simulink model "lazo_abierto"  (R2021b)
settings: Solver=VariableStepAuto  StartTime=0.0  StopTime=500  RelTol=1e-3
settings Model: Creator=sebas  LastModifiedBy=sebas

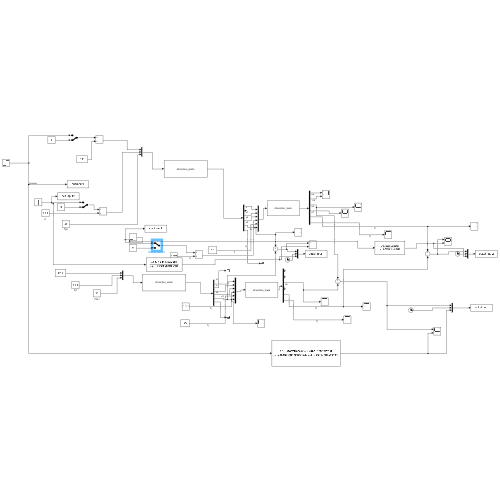
[thumbnail: Simulink's stored preview of the top-level diagram]
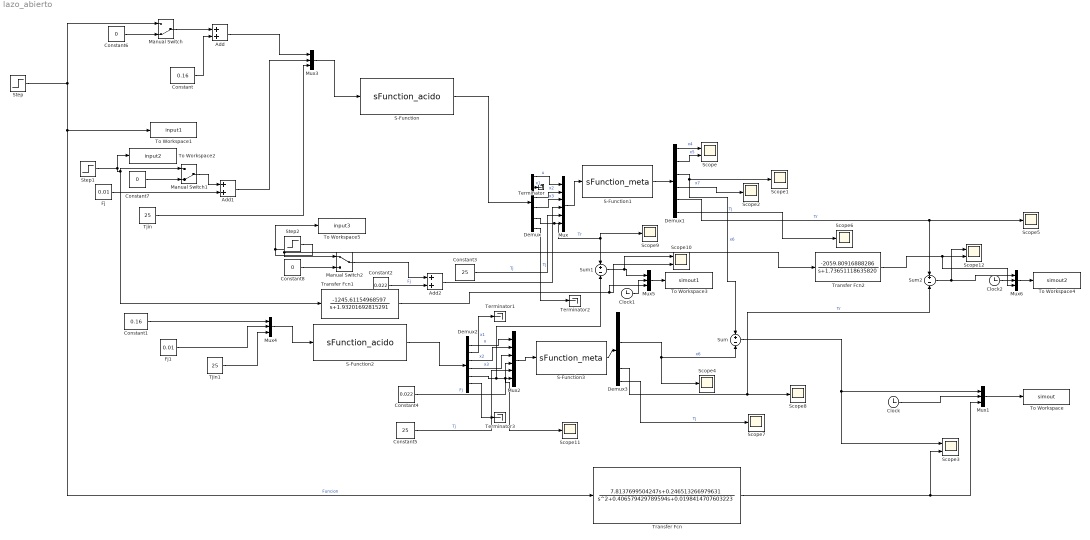
== system lazo_abierto ==
  Add : Sum
  Add1 : Sum
  Add2 : Sum
  Clock : Clock
  Clock1 : Clock
  Clock2 : Clock
  Constant : Constant  Value=0.16
  Constant1 : Constant  Value=0.16
  Constant2 : Constant  Value=0.022
  Constant3 : Constant  Value=25
  Constant4 : Constant  Value=0.022
  Constant5 : Constant  Value=25
  Constant6 : Constant  Value=0
  Constant7 : Constant  Value=0
  Constant8 : Constant  Value=0
  Demux{,1..3} (4 alike) : Demux  Outputs=6
  Fj : Constant  Value=0.01
  Fj1 : Constant  Value=0.01
  Manual Switch : ManualSwitch  CurrentSetting=0
  Manual Switch1 : ManualSwitch  CurrentSetting=0
  Manual Switch2 : ManualSwitch
  Mux : Mux  Inputs=6
  Mux{1,3..6} (5 alike) : Mux  Inputs=3
  Mux2 : Mux  Inputs=6
  S-Function : S-Function  FunctionName=sFunction_acido  SFunctionDeploymentMode=off  EnableBusSupport=off
  S-Function1 : S-Function  FunctionName=sFunction_meta  SFunctionDeploymentMode=off  EnableBusSupport=off
  S-Function2 : S-Function  FunctionName=sFunction_acido  SFunctionDeploymentMode=off  EnableBusSupport=off
  S-Function3 : S-Function  FunctionName=sFunction_meta  SFunctionDeploymentMode=off  EnableBusSupport=off
  Scope{,3,10,12} (4 alike) : Scope  NumInputPorts=2
  Scope{1..2,4..9,11} (9 alike) : Scope
  Step : Step  Time=150  After=0.5*0.16  SampleTime=0
  Step1 : Step  Time=150  After=0.01*0.5  SampleTime=0
  Step2 : Step  Time=150  After=0.0022 *0.5  SampleTime=0
  Sum : Sum  Inputs=+-
  Sum1 : Sum  Inputs=+-
  Sum2 : Sum  Inputs=+-
  Terminator{,1..3} (4 alike) : Terminator
  Tjin : Constant  Value=25
  Tjin1 : Constant  Value=25
  To Workspace : ToWorkspace  VariableName=simout  SampleTime=0.1
  To Workspace1 : ToWorkspace  VariableName=input1  SampleTime=0.1
  To Workspace2 : ToWorkspace  VariableName=input2  SampleTime=0.1
  To Workspace3 : ToWorkspace  VariableName=simout1  SampleTime=0.1
  To Workspace4 : ToWorkspace  VariableName=simout2  SampleTime=0.1
  To Workspace5 : ToWorkspace  VariableName=input3  SampleTime=0.1
  Transfer Fcn : TransferFcn  Numerator=[7.8137699504247 0.246513266979631]  Denominator=[1 0.406579429789594 0.0198414707603223]
  Transfer Fcn1 : TransferFcn  Numerator=[-1245.61154968597]  Denominator=[1 1.93201692815291]
  Transfer Fcn2 : TransferFcn  Numerator=[-2059.80916888286]  Denominator=[1 1.73651118635820]
  wires:
  Mux/1 -> S-Function1/1
  Demux1/4 -> Scope2/1  "x7"
  Demux1/3 -> Sum/1, Scope1/1  "x6"
  Demux1/2 -> Scope/2  "x5"
  Demux1/1 -> Scope/1  "x4"
  S-Function/1 -> Demux/1
  S-Function1/1 -> Demux1/1
  Constant/1 -> Add/2
  Add/1 -> Mux3/1
  Clock/1 -> Mux1/2
  Mux1/1 -> To Workspace/1
  Step/1 -> Transfer Fcn/1, To Workspace1/1, Manual Switch/1  "Funcion"
  Constant1/1 -> Mux4/1
  S-Function3/1 -> Demux3/1
  S-Function2/1 -> Demux2/1
  Mux2/1 -> S-Function3/1
  Demux3/3 -> Scope4/1, Sum/2  "x6"
  Sum/1 -> Mux1/1, Scope3/1
  Demux/1 -> Mux/1  "u"
  Demux/4 -> Mux/3  "x3"
  Demux/3 -> Mux/2  "x2"
  Demux/2 -> Terminator/1  "x1"
  Demux2/4 -> Mux2/3  "x3"
  Demux2/3 -> Mux2/2  "x2"
  Demux2/1 -> Mux2/1  "u"
  Demux2/2 -> Terminator1/1  "x1"
  Fj/1 -> Add1/2
  Tjin/1 -> Mux3/3
  Mux3/1 -> S-Function/1
  Demux/5 -> Scope9/1, Sum1/1, Mux/6  "Tr"
  Demux/6 -> Terminator2/1  "Tj"
  Constant2/1 -> Add2/2  "Fj"
  Constant3/1 -> Mux/5  "Tj"
  Demux1/5 -> Scope5/1, Sum2/1  "Tr"
  Demux1/6 -> Scope6/1  "Tj"
  Tjin1/1 -> Mux4/3
  Fj1/1 -> Mux4/2
  Mux4/1 -> S-Function2/1
  Demux2/6 -> Terminator3/1
  Constant4/1 -> Mux2/4  "Fj"
  Constant5/1 -> Mux2/5  "Tj"
  Demux3/6 -> Scope7/1  "Tj"
  Demux3/5 -> Sum2/2, Scope8/1  "Tr"
  Step1/1 -> Transfer Fcn1/1, Manual Switch1/1, To Workspace2/1
  Add1/1 -> Mux3/2
  Transfer Fcn/1 -> Mux1/3, Scope3/2
  Manual Switch/1 -> Add/1
  Constant6/1 -> Manual Switch/2
  Sum1/1 -> Scope10/1, Mux5/1
  Clock1/1 -> Mux5/2
  Mux5/1 -> To Workspace3/1
  Manual Switch1/1 -> Add1/1
  Constant7/1 -> Manual Switch1/2
  Constant8/1 -> Manual Switch2/2
  Step2/1 -> To Workspace5/1, Manual Switch2/1, Transfer Fcn2/1
  Manual Switch2/1 -> Add2/1
  Add2/1 -> Mux/4
  Clock2/1 -> Mux6/2
  Mux6/1 -> To Workspace4/1
  Transfer Fcn1/1 -> Mux5/3, Scope10/2
  Demux2/5 -> Sum1/2, Scope11/1, Mux2/6
  Sum2/1 -> Scope12/1, Mux6/1
  Transfer Fcn2/1 -> Mux6/3, Scope12/2
